simulink model "adaptive_sonar_system"  (R2026a)
settings: Solver=FixedStepDiscrete  StopTime=0.045  FixedStep=2.5e-7
libraries: simulink x4
settings Model: Creator=harsh  LastModifiedBy=harsh

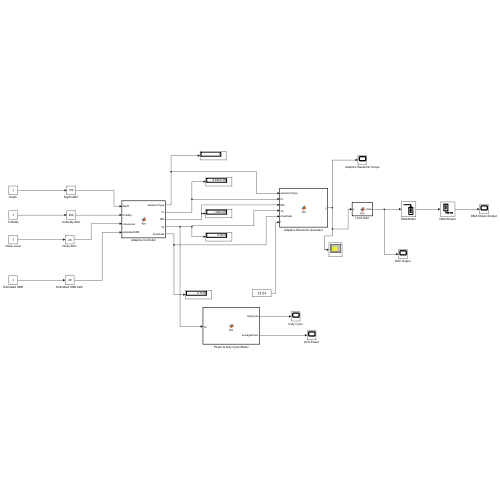
[thumbnail: Simulink's stored preview of the top-level diagram]
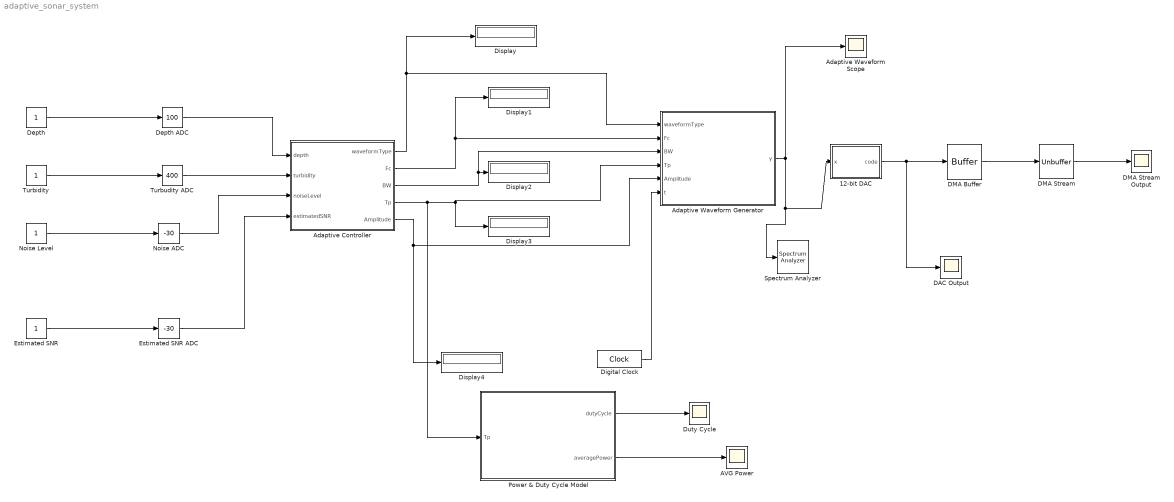
== system adaptive_sonar_system ==
  12-bit DAC : MATLAB Function  TreatAsAtomicUnit=on
  AVG Power : Scope
      settings: ActiveDisplayYMinimum=0.35  ActiveDisplayYMaximum=0.54999999999999993  DataLoggingVariableName=ScopeData4
  Adaptive Controller : MATLAB Function  TreatAsAtomicUnit=on
  Adaptive Waveform Generator : MATLAB Function  TreatAsAtomicUnit=on
  Adaptive Waveform Scope : Scope
      settings: ActiveDisplayYMinimum=-1.1238475211281447  ActiveDisplayYMaximum=1.0105235726218558  DataLoggingVariableName=ScopeData2
  DAC Output : Scope
      settings: ActiveDisplayYMinimum=1725.8049877841772  ActiveDisplayYMaximum=3886.8644916637541
  DMA Buffer : Buffer  N=8000  OutputFrames=off
  DMA Stream : Unbuffer
  DMA Stream Output : Scope
      settings: ActiveDisplayYMinimum=-476.49183976423546  ActiveDisplayYMaximum=7442.0186322909785
  Depth : Constant
  Depth ADC : simulink/Math Operations/Slider Gain  gain=100  low=0  high=200
  Digital Clock : DigitalClock  SampleTime=5e-7
  Display{,1..4} (5 alike) : Display
  Duty Cycle : Scope
      settings: ActiveDisplayYMinimum=0.078987893081761  ActiveDisplayYMaximum=0.101037893081761  DataLoggingVariableName=ScopeData3
  Estimated SNR : Constant
  Estimated SNR ADC : simulink/Math Operations/Slider Gain  gain=-30  low=-40  high=10
  Noise ADC : simulink/Math Operations/Slider Gain  gain=-30  low=-40  high=0
  Noise Level : Constant
  Power & Duty Cycle Model : MATLAB Function  TreatAsAtomicUnit=on
  Spectrum Analyzer : SpectrumAnalyzer  WindowPosition=[577.000000,212.000000,800.000000,500.000000,]  ScopeFrameLocation=window  SampleRateSource=Property  SampleRate=4000000  WindowInvariantSamplesPerUpdate=on  Span=4000000  StartFrequency=-2000000  StopFrequency=2000000  YLimits=[-57.6699 15.3749]
  Turbidity : Constant
  Turbudity ADC : simulink/Math Operations/Slider Gain  gain=400  low=0  high=1000
  wires:
  Depth/1 -> Depth ADC/1
  Turbidity/1 -> Turbudity ADC/1
  Noise Level/1 -> Noise ADC/1
  Estimated SNR/1 -> Estimated SNR ADC/1
  Adaptive Controller/1(waveformType) -> Adaptive Waveform Generator/1(waveformType), Display/1
  Adaptive Controller/2(Fc) -> Adaptive Waveform Generator/2(Fc), Display1/1
  Adaptive Controller/3(BW) -> Adaptive Waveform Generator/3(BW), Display2/1
  Adaptive Controller/4(Tp) -> Adaptive Waveform Generator/4(Tp), Display3/1, Power & Duty Cycle Model/1(Tp)
  Adaptive Controller/5(Amplitude) -> Display4/1, Adaptive Waveform Generator/5(Amplitude)
  Adaptive Waveform Generator/1(y) -> Adaptive Waveform Scope/1, 12-bit DAC/1(x), Spectrum Analyzer/1
  Digital Clock/1 -> Adaptive Waveform Generator/6(t)
  12-bit DAC/1(code) -> DAC Output/1, DMA Buffer/1
  DMA Buffer/1 -> DMA Stream/1
  DMA Stream/1 -> DMA Stream Output/1
  Depth ADC/1 -> Adaptive Controller/1(depth)
  Turbudity ADC/1 -> Adaptive Controller/2(turbidity)
  Noise ADC/1 -> Adaptive Controller/3(noiseLevel)
  Estimated SNR ADC/1 -> Adaptive Controller/4(estimatedSNR)
  Power & Duty Cycle Model/1(dutyCycle) -> Duty Cycle/1
  Power & Duty Cycle Model/2(averagePower) -> AVG Power/1

== matlab function adaptive_sonar_system/Adaptive Waveform Generator ==
  data: waveformType input; y output; Fc input; BW input; Tp input; Amplitude input; t input
function y = fcn(waveformType,Fc,BW,Tp,Amplitude,t)

% =========================================================
% SIH 26058 - ADAPTIVE WAVEFORM GENERATOR PoC
% =========================================================

PRI = 20e-3;

% Position inside current PRI
tau = mod(t,PRI);

% Default output
y = 0;

% Generate only during pulse
if tau < Tp

    % ---------------------------------------------
    % LFM CHIRP
    % ---------------------------------------------
    if waveformType == 1

        fStart = Fc - BW/2;
        k = BW/Tp;

        phase = 2*pi*(fStart*tau + 0.5*k*tau^2);

        y = Amplitude * sin(phase);

        % ---------------------------------------------
        % GEOMETRIC SWEEP
        % ---------------------------------------------
    elseif waveformType == 2

        fStart = max(1e3,Fc - BW/2);
        fEnd   = Fc + BW/2;

        ratio = fEnd/fStart;

        phase = 2*pi*fStart*Tp/log(ratio) * ...
            (exp((tau/Tp)*log(ratio))-1);

        y = Amplitude * sin(phase);

        % ---------------------------------------------
        % PHASE-CODED PULSE
        % ---------------------------------------------
    elseif waveformType == 3

        chipCount = 8;

        chipTime = Tp/chipCount;

        chipIndex = floor(tau/chipTime);

        % Simple alternating phase code
        if mod(chipIndex,2) == 0
            phaseSign = 1;
        else
            phaseSign = -1;
        end

        y = Amplitude * phaseSign * sin(2*pi*Fc*tau);

    end

    % ---------------------------------------------
    % HANN WINDOW
    % ---------------------------------------------
    window = 0.5*(1-cos(2*pi*tau/Tp));

    y = y * window;

end

end

== matlab function adaptive_sonar_system/Adaptive Controller ==
  data: depth input; waveformType output; turbidity input; noiseLevel input; estimatedSNR input; Fc output; BW output; Tp output; Amplitude output
function [waveformType,Fc,BW,Tp,Amplitude] = fcn( ...
    depth,turbidity,noiseLevel,estimatedSNR)

% =========================================================
% SIH 26058 - ADAPTIVE SONAR PoC CONTROLLER
% Slider-responsive digital twin
% =========================================================

% ----------- LIMIT INPUTS -----------
depth        = max(0,min(200,depth));
turbidity    = max(0,min(1000,turbidity));
noiseLevel   = max(-40,min(0,noiseLevel));
estimatedSNR = max(-40,min(10,estimatedSNR));

% =========================================================
% DEPTH -> CENTER FREQUENCY
% Shallow  : higher frequency
% Deep     : lower frequency
% =========================================================

Fc = 425e3 - (depth/200)*265e3;

% =========================================================
% TURBIDITY -> BANDWIDTH
% Higher turbidity -> narrower bandwidth
% =========================================================

BW = 200e3 - (turbidity/1000)*80e3;

% =========================================================
% NOISE -> AMPLITUDE
% Higher noise -> higher transmit amplitude
% =========================================================

Amplitude = 0.65 + ((noiseLevel + 40)/40)*0.35;

% =========================================================
% SNR -> PULSE DURATION
% Lower SNR -> longer pulse
% =========================================================

Tp = 1e-3 + ((10-estimatedSNR)/50)*1e-3;

% =========================================================
% WAVEFORM TYPE
% =========================================================

if estimatedSNR < -25
    waveformType = 3;       % Phase-coded

elseif estimatedSNR < -10
    waveformType = 2;       % Geometric sweep

else
    waveformType = 1;       % LFM
end

% =========================================================
% SAFETY LIMITS
% =========================================================

Fc = max(160e3,min(425e3,Fc));

BW = max(120e3,min(200e3,BW));

Tp = max(1e-3,min(2e-3,Tp));

Amplitude = max(0.65,min(1.0,Amplitude));

end

== matlab function adaptive_sonar_system/12-bit DAC ==
  data: x input; code output
function code = fcn(x)
% SIH 26058
% 12-bit DAC Quantization
%
% Input:
%   x = normalized waveform [-1, +1]
%
% Output:
%   code = 12-bit DAC code [0, 4095]

DAC_MAX = 4095;
DAC_MID = 2048;

% Limit input to valid normalized range
x = min(max(x, -1), 1);

% Convert bipolar waveform to unipolar DAC code
code = round(DAC_MID + 2047*x);

% Safety saturation
code = min(max(code, 0), DAC_MAX);

% 12-bit DAC data stored as uint16
code = uint16(code);

end

== matlab function adaptive_sonar_system/Power & Duty Cycle Model ==
  data: Tp input; dutyCycle output; averagePower output
function [dutyCycle,averagePower] = fcn(Tp)

% =========================================================
% SIH 26058 - PoC POWER / DUTY-CYCLE MODEL
% =========================================================

PRI = 20e-3;      % 20 ms PRI
activePower = 5;  % 5 W during transmission

% Duty cycle
dutyCycle = Tp / PRI;

% Average power
averagePower = activePower * dutyCycle;

end
